simulink model "robot_model_linear_final"  (R2024b)
settings: Solver=VariableStepAuto  StartTime=0.0  StopTime=20.0  RelTol=1e-3
model workspace (MAT data in the model file):
  pitchd = Simulink.Parameter
  pitchd.Value = 1
  pitchd.Complexity = 'real'
  pitchd.Dimensions = [1 1]
  pitchd.DataType = 'auto'
  yawd = Simulink.Parameter
  yawd.Value = 1
  yawd.Complexity = 'real'
  yawd.Dimensions = [1 1]
  yawd.DataType = 'auto'
values from neighbouring files (symbols this model uses):
  A = [0   1.0000        0        0 ... (first row only)    [invgui.m]    (also in p1.m = 14; p2.m = 14; robot.m = [0 1 0 0; robot_cascade.m = [ 0, 1, 0, 0)
  B = [0; 1.8182; 0; 4.5455]    [invgui.m]    (also in p1.m = 18; p2.m = 18; robot.m = [0; 1/M; 0; 1/(l*M)] / R; robot_cascade.m = B ./ r_wheel)
  C = [1 0 0 0]    [invgui.m]    (also in p1.m = 10; p2.m = 10; robot.m = eye(4); robot_cascade.m = [ 1 0 0 0; 0 0 1 0;])
  D = (K.Kp * KpMultiplier) + (K.Ki * KiMultiplier / s) + (K.Kd * KdMultiplier * -p * s / (s - p))    [Ktune.m]    (also in findZeros.m = (s-Z(1))*(s-Z(2))/(Z(1)*Z(2))*Dp; invgui.m = [0]; p1.m = 18; p2.m = 18)
  Km = 16.129/1000    (= 0.016129)    [robot.m]    (also in robot_cascade.m = 16.1290322581; robot_linear.m = 0.212207; robot_lqr.m = 0.212207)
  n = 18.75    [robot.m]    (also in robot_cascade.m; robot_linear.m; robot_lqr.m)
  R = 1    [invgui.m]    (also in robot.m = 0.04; robot_lqr.m = 200)
libraries: cstblocks x8, slpidlib x2
settings Model: Creator=cosr3  LastModifiedBy=cosr3

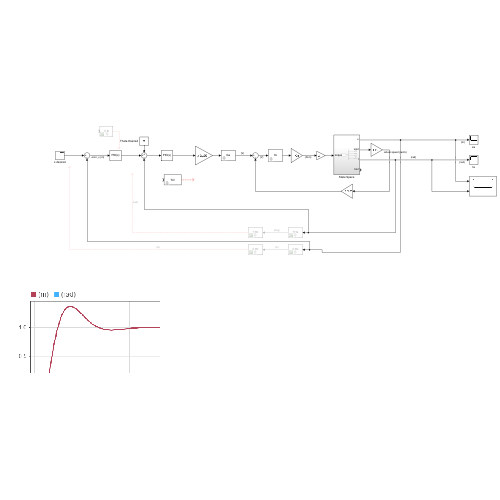
[thumbnail: Simulink's stored preview of the top-level diagram]
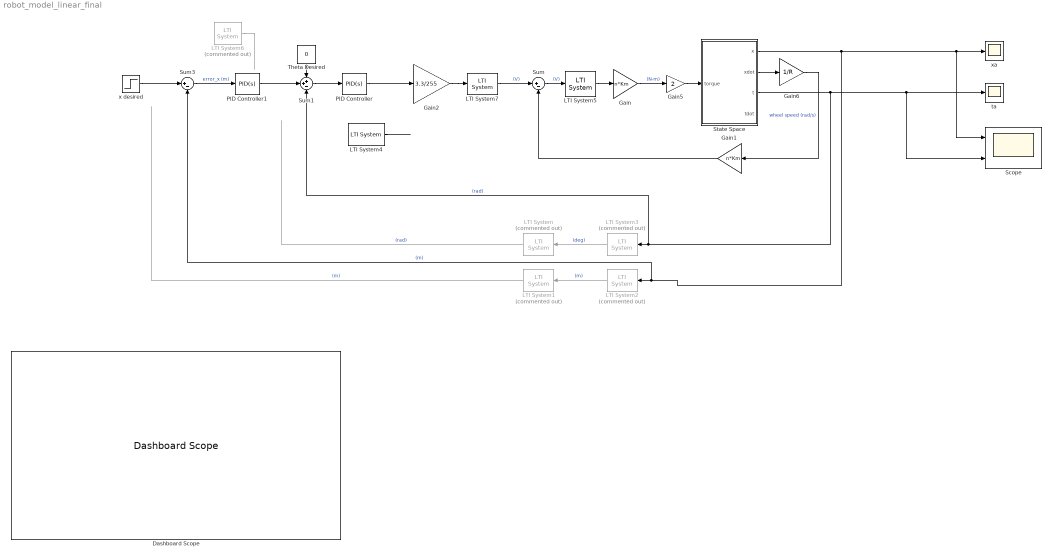
== system robot_model_linear_final ==
  Dashboard Scope : DashboardScope
  Gain : Gain  Gain=n*Km
  Gain1 : Gain  Gain=n*Km
  Gain2 : Gain  Gain=3.3/255
  Gain5 : Gain  Gain=2
  Gain6 : Gain  Gain=1/R
  LTI System : cstblocks/LTI System  Commented=on  sys=T.Hc  IC=[]  PadeOrder=0
  LTI System1 : cstblocks/LTI System  Commented=on  sys=X.Hc  IC=[]  PadeOrder=0
  LTI System2 : cstblocks/LTI System  Commented=on  sys=X.Hs  IC=[]  PadeOrder=0
  LTI System3 : cstblocks/LTI System  Commented=on  sys=T.Hs  IC=[]  PadeOrder=0
  LTI System4 : cstblocks/LTI System  sys=T.D  IC=[]  PadeOrder=0
  LTI System5 : cstblocks/LTI System  sys=Ye  IC=[]  PadeOrder=0
  LTI System6 : cstblocks/LTI System  Commented=on  sys=X.D  IC=[]  PadeOrder=0
  LTI System7 : cstblocks/LTI System  sys=Ga  IC=[]  PadeOrder=0
  PID Controller : slpidlib/PID Controller  Controller=PID  Form=Parallel  TimeDomain=Continuous-time  UseExternalTs=off  SampleTime=-1  IntegratorMethod=Forward Euler  FilterMethod=Forward Euler  ControllerParametersSource=internal  P=3200  I=12000  UseKiTs=off  D=300  UseExternalDerivativeSource=off  N=4700  UseFilter=on  TunerSelectOption=Transfer Function Based (PID Tuner App)  InitialConditionSource=internal  InitialConditionForIntegrator=0  InitialConditionForFilter=0  DifferentiatorICPrevScaledInput=0  ExternalReset=none  TrackingMode=off  Kt=1  LimitOutput=off  SatLimitsSource=internal  UpperSaturationLimit=inf  LowerSaturationLimit=-inf  LinearizeAsGain=on  AntiWindupMode=none  Kb=1  LimitIntegrator=off  UpperIntegratorSaturationLimit=inf  LowerIntegratorSaturationLimit=-inf  POutMin=[]  POutMax=[]  IOutMin=[]  IOutMax=[]  DOutMin=[]  DOutMax=[]  NOutMin=[]  NOutMax=[]  SumOutMin=[]  SumOutMax=[]  SaturationOutMin=[]  SaturationOutMax=[]  PParamMin=[]  PParamMax=[]  IParamMin=[]  IParamMax=[]  DParamMin=[]  DParamMax=[]  NParamMin=[]  NParamMax=[]  KbParamMin=[]  KbParamMax=[]  KtParamMin=[]  KtParamMax=[]  KbOutMin=[]  KbOutMax=[]  KtOutMin=[]  KtOutMax=[]  IntegratorOutMin=[]  IntegratorOutMax=[]  FilterOutMin=[]  FilterOutMax=[]  SumI1OutMin=[]  SumI1OutMax=[]  SumI2OutMin=[]  SumI2OutMax=[]  SumI3OutMin=[]  SumI3OutMax=[]  SumI4OutMin=[]  SumI4OutMax=[]  SumDOutMin=[]  SumDOutMax=[]  DifferentiatorOutMin=[]  DifferentiatorOutMax=[]  FilterDiffOutCoefMin=[]  FilterDiffOutCoefMax=[]  ReciprocalOutMin=[]  ReciprocalOutMax=[]  SumDenOutMin=[]  SumDenOutMax=[]  SumNumOutMin=[]  SumNumOutMax=[]  DivideOutMin=[]  DivideOutMax=[]  UdiffTsProdOutMin=[]  UdiffTsProdOutMax=[]  NTsProdOutMin=[]  NTsProdOutMax=[]  UintegralTsProdOutMin=[]  UintegralTsProdOutMax=[]  UngainTsProdOutMin=[]  UngainTsProdOutMax=[]  ClampingZeroOutDataTypeStr=Inherit: Inherit via back propagation  ClampingZeroOutMin=[]  ClampingZeroOutMax=[]  FilterDenConstantOutDataTypeStr=Inherit: Inherit via back propagation  FilterDenConstantOutMin=[]  FilterDenConstantOutMax=[]  PCopyOutDataTypeStr=Inherit: Inherit via back propagation  PCopyOutMin=[]  PCopyOutMax=[]  NCopyOutDataTypeStr=Inherit: Inherit via back propagation  NCopyOutMin=[]  NCopyOutMax=[]  IntegratorContinuousStateAttributes=''  IntegratorStateMustResolveToSignalObject=off  IntegratorRTWStateStorageClass=Auto  FilterContinuousStateAttributes=''  FilterStateMustResolveToSignalObject=off  FilterRTWStateStorageClass=Auto  ParallelPVariant=InternalParameters  IdealPVariant=Disabled  IVariant=InternalParameters  DVariant=InternalParameters  IntegratorVariant=Continuous  SatVariant=Disabled  AWVariant=Passthrough  PCopyVariant=Disabled  TRVariant=Disabled  FdbkBlocksVariant=Forward  IdealPFdbkVariant=Disabled  SatFdbkVariant=Disabled  DerivativeFilterVariant=ContFilter  NVariant=InternalParameters  NCopyVariant=Disabled  FilterICVariant=InternalICsFilter  IntegratorICVariant=InternalICs  ExternalResetVariant=Disabled  TRSumVariant=Passthrough  SumFdbkVariant=Disabled  SumVariant=Sum_PID  TsampFilterVariant=InternalTs  TsampNgainVariant=Passthrough  TsampIntegralVariant=Disabled_SignalSpec  ExternalSaturationOutDataTypeStr=Inherit: Same as second input  DerivativeSourceVariant=ErrorSignal  PreIntVariant=InternalPreInt
  PID Controller1 : slpidlib/PID Controller  Controller=PID  Form=Parallel  TimeDomain=Continuous-time  UseExternalTs=off  SampleTime=-1  IntegratorMethod=Forward Euler  FilterMethod=Forward Euler  ControllerParametersSource=internal  P=-0.065  I=-0.00285  UseKiTs=off  D=-0.08  UseExternalDerivativeSource=off  N=5  UseFilter=on  TunerSelectOption=Transfer Function Based (PID Tuner App)  InitialConditionSource=internal  InitialConditionForIntegrator=0  InitialConditionForFilter=0  DifferentiatorICPrevScaledInput=0  ExternalReset=none  TrackingMode=off  Kt=1  LimitOutput=off  SatLimitsSource=internal  UpperSaturationLimit=inf  LowerSaturationLimit=-inf  LinearizeAsGain=on  AntiWindupMode=none  Kb=1  LimitIntegrator=off  UpperIntegratorSaturationLimit=inf  LowerIntegratorSaturationLimit=-inf  POutMin=[]  POutMax=[]  IOutMin=[]  IOutMax=[]  DOutMin=[]  DOutMax=[]  NOutMin=[]  NOutMax=[]  SumOutMin=[]  SumOutMax=[]  SaturationOutMin=[]  SaturationOutMax=[]  PParamMin=[]  PParamMax=[]  IParamMin=[]  IParamMax=[]  DParamMin=[]  DParamMax=[]  NParamMin=[]  NParamMax=[]  KbParamMin=[]  KbParamMax=[]  KtParamMin=[]  KtParamMax=[]  KbOutMin=[]  KbOutMax=[]  KtOutMin=[]  KtOutMax=[]  IntegratorOutMin=[]  IntegratorOutMax=[]  FilterOutMin=[]  FilterOutMax=[]  SumI1OutMin=[]  SumI1OutMax=[]  SumI2OutMin=[]  SumI2OutMax=[]  SumI3OutMin=[]  SumI3OutMax=[]  SumI4OutMin=[]  SumI4OutMax=[]  SumDOutMin=[]  SumDOutMax=[]  DifferentiatorOutMin=[]  DifferentiatorOutMax=[]  FilterDiffOutCoefMin=[]  FilterDiffOutCoefMax=[]  ReciprocalOutMin=[]  ReciprocalOutMax=[]  SumDenOutMin=[]  SumDenOutMax=[]  SumNumOutMin=[]  SumNumOutMax=[]  DivideOutMin=[]  DivideOutMax=[]  UdiffTsProdOutMin=[]  UdiffTsProdOutMax=[]  NTsProdOutMin=[]  NTsProdOutMax=[]  UintegralTsProdOutMin=[]  UintegralTsProdOutMax=[]  UngainTsProdOutMin=[]  UngainTsProdOutMax=[]  ClampingZeroOutDataTypeStr=Inherit: Inherit via back propagation  ClampingZeroOutMin=[]  ClampingZeroOutMax=[]  FilterDenConstantOutDataTypeStr=Inherit: Inherit via back propagation  FilterDenConstantOutMin=[]  FilterDenConstantOutMax=[]  PCopyOutDataTypeStr=Inherit: Inherit via back propagation  PCopyOutMin=[]  PCopyOutMax=[]  NCopyOutDataTypeStr=Inherit: Inherit via back propagation  NCopyOutMin=[]  NCopyOutMax=[]  IntegratorContinuousStateAttributes=''  IntegratorStateMustResolveToSignalObject=off  IntegratorRTWStateStorageClass=Auto  FilterContinuousStateAttributes=''  FilterStateMustResolveToSignalObject=off  FilterRTWStateStorageClass=Auto  ParallelPVariant=InternalParameters  IdealPVariant=Disabled  IVariant=InternalParameters  DVariant=InternalParameters  IntegratorVariant=Continuous  SatVariant=Disabled  AWVariant=Passthrough  PCopyVariant=Disabled  TRVariant=Disabled  FdbkBlocksVariant=Forward  IdealPFdbkVariant=Disabled  SatFdbkVariant=Disabled  DerivativeFilterVariant=ContFilter  NVariant=InternalParameters  NCopyVariant=Disabled  FilterICVariant=InternalICsFilter  IntegratorICVariant=InternalICs  ExternalResetVariant=Disabled  TRSumVariant=Passthrough  SumFdbkVariant=Disabled  SumVariant=Sum_PID  TsampFilterVariant=InternalTs  TsampNgainVariant=Passthrough  TsampIntegralVariant=Disabled_SignalSpec  ExternalSaturationOutDataTypeStr=Inherit: Same as second input  DerivativeSourceVariant=ErrorSignal  PreIntVariant=InternalPreInt
  Scope : Scope  NumInputPorts=2
  State Space : Subsystem
  Sum : Sum  Inputs=|+-
  Sum1 : Sum  Inputs=++-
  Sum3 : Sum  Inputs=|+-
  Theta Desired : Constant  Value=0
  ta : Scope
  x desired : Step  SampleTime=0
  xa : Scope
  wires:
  LTI System5/1 -> Gain/1
  Gain/1 -> Gain5/1  "(N-m)"
  LTI System3/1 -> LTI System/1  "(deg)"
  LTI System2/1 -> LTI System1/1  "(m)"
  Sum/1 -> LTI System5/1  "(V)"
  Gain1/1 -> Sum/2
  LTI System7/1 -> Sum/1  "(V)"
  x desired/1 -> Sum3/1
  LTI System/1 -> ?  "(rad)"
  LTI System1/1 -> ?  "(m)"
  Gain2/1 -> LTI System7/1
  State Space/1(x) -> Scope/1, xa/1, Sum3/2, LTI System2/1  "(m)"
  State Space/3(t) -> Sum1/3, LTI System3/1, Scope/2, ta/1  "(rad)"
  State Space/2(xdot) -> Gain6/1
  Gain6/1 -> Gain1/1  "wheel speed (rad/s)"
  Sum3/1 -> PID Controller1/1  "error_x (m)"
  Gain5/1 -> State Space/1(torque)
  Theta Desired/1 -> Sum1/1
  LTI System4/1 -> ?
  Sum1/1 -> PID Controller/1
  LTI System6/1 -> ?
  PID Controller/1 -> Gain2/1
  PID Controller1/1 -> Sum1/2

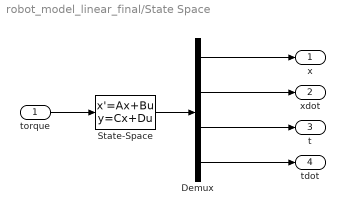
== system robot_model_linear_final/State Space ==
  torque : Inport
  Demux : Demux
  State-Space : StateSpace  A=A  B=B  C=C  D=D  InitialCondition=0  ContinuousStateAttributes='state'
  x : Outport
  xdot : Outport  Port=2
  t : Outport  Port=3
  tdot : Outport  Port=4
  wires:
  Demux/1 -> x/1
  State-Space/1 -> Demux/1
  Demux/4 -> tdot/1
  Demux/2 -> xdot/1
  torque/1 -> State-Space/1
  Demux/3 -> t/1
